simulink model "Multicopter_vPC"  (R2021a)
settings: Solver=ode4  StartTime=0.0  StopTime=inf  FixedStep=0.0002  RelTol=1e-3
values from neighbouring files (symbols this model uses):
  ModelFailBatt_CustomHovTime = 15    [Init.m]
  ModelFailBatt_isEnable = boolean(0)    [Init.m]
  ModelFailBatt_islowCapacity = boolean(0)    [Init.m]
  ModelFailBatt_isLowVoltage = boolean(0)    [Init.m]
  ModelFailBatt_isPowOff = boolean(0)    [Init.m]
  ModelFailBatt_isUseCustomHovTime = boolean(0)    [Init.m]
  ModelFailBatt_remainCapacityRatio = 0.2    [Init.m]
  ModelFailBatt_remainVoltageRatio = 0.5    [Init.m]
  ModelFailEnable = boolean(0)    [Init.m]
  ModelFailLoad_isEnable = boolean(0)    [Init.m]
  ModelFailLoad_isLoadFall = boolean(0)    [Init.m]
  ModelFailLoad_isLoadLeak = boolean(0)    [Init.m]
  ModelFailLoad_isLoadShift = boolean(0)    [Init.m]
  ModelFailLoad_LoadLeakRatioRate = 0    [Init.m]
  ModelFailLoad_loadMassRatio = 0    [Init.m]
  ModelFailLoad_LoadShiftXRatio = 0    [Init.m]
  ModelFailLoad_LoadShiftYRatio = 0    [Init.m]
  ModelFailLoad_LoadShiftZRatio = 0    [Init.m]
  ModelFailProp_isEnable = boolean(1)    [Init.m]
  ModelFailProp_PropEffRatioVec = ones(1,8)    [Init.m]
  ModelFailWind_ConstWindX = 0    [Init.m]
  ModelFailWind_ConstWindY = 0    [Init.m]
  ModelFailWind_ConstWindZ = 0    [Init.m]
  ModelFailWind_GustWindFreq = 0    [Init.m]
  ModelFailWind_GustWindStrength = 0    [Init.m]
  ModelFailWind_isConstWind = boolean(0)    [Init.m]
  ModelFailWind_isEnable = boolean(0)    [Init.m]
  ModelFailWind_isGustWind = boolean(0)    [Init.m]
  ModelFailWind_isSheerWind = boolean(0)    [Init.m]
  ModelFailWind_isTurbWind = boolean(0)    [Init.m]
  ModelFailWind_SheerWindDirec = 0    [Init.m]
  ModelFailWind_SheerWindStrength = 0    [Init.m]
  ModelFailWind_TurbWindDirec = 0    [Init.m]
  ModelFailWind_TurbWindStrength = 0    [Init.m]
  ModelInit_RPM = 0    [Init.m]
  ModelParam_BattHoverMinutes = 18    [Init.m]
  ModelParam_BattHoverThr = 0.609    [Init.m]
  ModelParam_envAltitude = -41.5260009765625    (= -41.5260009766)    [Init.m]
  ModelParam_GlobalNoiseGainSwitch = 0    [Init.m]
  ModelParam_GPSEphFinal = 0.3    [Init.m]
  ModelParam_GPSEpvFinal = 0.4    [Init.m]
  ModelParam_GPSFix3DFix = 3    [Init.m]
  ModelParam_GPSSatsVisible = 10    [Init.m]
  ModelParam_motorCr = 1148    [Init.m]
  ModelParam_motorJm = 0.0001287    [Init.m]
  ModelParam_motorMinThr = 0.05    [Init.m]
  ModelParam_motorT = 0.02    [Init.m]
  ModelParam_motorWb = -141.4    [Init.m]
  ModelParam_noiseBaroCoupleWithSpeed = 0    [Init.m]
  ModelParam_noiseGPSSampTime = 0.2    [Init.m]
  ModelParam_noisePowerIMU = 0    [Init.m]
  ModelParam_noisePowerOffGainAccel = 0.04    [Init.m]
  ModelParam_noisePowerOffGainAccelZ = 0.03    [Init.m]
  ModelParam_noisePowerOffGainGyro = 0.02    [Init.m]
  ModelParam_noisePowerOffGainGyroZ = 0.025    [Init.m]
  ModelParam_noisePowerOffGainMag = 0.02    [Init.m]
  ModelParam_noisePowerOffGainMagZ = 0.035    [Init.m]
  ModelParam_noisePowerOnGainAccel = 0.8    [Init.m]
  ModelParam_noisePowerOnGainAccelZ = 4.5    [Init.m]
  ModelParam_noisePowerOnGainGyro = 2    [Init.m]
  ModelParam_noisePowerOnGainGyroZ = 1    [Init.m]
  ModelParam_noisePowerOnGainMag = 0.025    [Init.m]
  ModelParam_noisePowerOnGainMagZ = 0.05    [Init.m]
  ModelParam_noiseSampleTimeAccel = 0.001    [Init.m]
  ModelParam_noiseSampleTimeGyro = 0.001    [Init.m]
  ModelParam_noiseSampleTimeMag = 0.01    [Init.m]
  ModelParam_noiseUpperBaro = 0    [Init.m]
  ModelParam_noiseUpperGPS = 0.5    [Init.m]
  ModelParam_noiseUpperWindBodyRatio = 0    [Init.m]
  ModelParam_noiseWindSampTime = 0.001    [Init.m]
  ModelParam_rotorCm = 1.779e-07    [Init.m]
  ModelParam_rotorCt = 1.105e-05    [Init.m]
  ModelParam_timeSampBaro = 0.01    [Init.m]
  ModelParam_uavCCm = [0.0035 0.0039 0.0034]    [Init.m]
  ModelParam_uavCd = 0.055    [Init.m]
  ModelParam_uavDearo = 0.12    [Init.m]
  ModelParam_uavJ = [ModelParam_uavJxx,0,0;     0,ModelParam_uavJyy,0;     0,0,ModelParam_uavJzz]    [Init.m]
  ModelParam_uavMass = 1.4    [Init.m]
  ModelParam_uavMotNumbs = int8(4)    [Init.m]
  ModelParam_uavR = 0.225    [Init.m]
  ModelParam_uavType = int8(3)    [Init.m]
undefined symbols (not defined in the file or in its folder): d_i, Earth, F, h_i, Light, MIL, ModelParam_GPSEphInitial, ModelParam_GPSEphTimeConstant, ModelParam_GPSEpvInitial, ModelParam_GPSEpvTimeConstant, ModelParam_noiseLowPassFilterCoeAccel, ModelParam_noiseLowPassFilterCoeGyro, ModelParam_timeSamp, Moderate, Newton, Raphson, WGS84
libraries: simulink x12, aerolibasang x4, aerolibwind2 x3, aerolibtransform2 x3, sharedtransform x3, aerolibutil x2, sharedutil x2, shared6dof x1, aerolibatmos2 x1, aerolibconvert2 x1, aerolibobsolete x1, aerolibnav x1
(part 1 of 3)
settings Model: SimulationMode=accelerator  Creator=Jinrui  LastModifiedBy=YeBobo
settings SolverCC: AlgebraicLoopSolver=TrustRegion
settings DataIOCC: SaveFormat=Structure  SaveOutput=off  SignalLogging=off  DSMLogging=off  SaveTime=off  ReturnWorkspaceOutputs=off
settings DebuggingCC: ParameterTunabilityLossMsg=error  RootOutportRequireBusObject=error  StrictBusMsg=ErrorOnBusTreatedAsVector  SFMachineParentedDataDiag=warning  ArithmeticOperatorsInVariantConditions=warning
settings HardwareCC: ProdBitPerPointer=32  ProdBitPerSizeT=32  ProdBitPerPtrDiffT=32  ProdLargestAtomicFloat=None  ProdWordSize=32  ProdHWDeviceType=Intel->x86/Pentium
settings SFSimCC: SimUseLocalCustomCode=off  CustomCodeUndefinedFunction=UseInterfaceOnly
settings RTWCC: Description=NI Phar Lap Real-Time & Windows Targets  SystemTargetFile=NIVeriStand.tlc  PackageName=MulticopterModel  TemplateMakefile=NIVeriStand_vc.tmf  GenerateReport=on  RTWUseLocalCustomCode=off  LaunchReport=on
settings CodeAppCC: ForceParamTrailComments=on  OperatorAnnotations=on  StateflowObjectComments=on  MATLABSourceComments=on
settings STFCustomTargetCC: TargetLangStandard=C99 (ISO)  MatFileLogging=on  MATLABClassNameForMDSCustomization=Simulink.SoftwareTarget.TargetSpecificTriggerConfigurationBase  UseToolchainInfoCompliant=off  SystemTargetFile=NIVeriStand.tlc
settings GRTTargetCC: ParMdlRefBuildCompliant=off  CompOptLevelCompliant=off  ConcurrentExecutionCompliant=off  CombineOutputUpdateFcns=off  MATLABClassNameForMDSCustomization=Simulink.SoftwareTarget.TargetSpecificTriggerConfigurationBase  CPPClassGenCompliant=off  GRTInterface=on  UseToolchainInfoCompliant=off
settings SimscapeCC: SimscapeNormalizeSystem=off

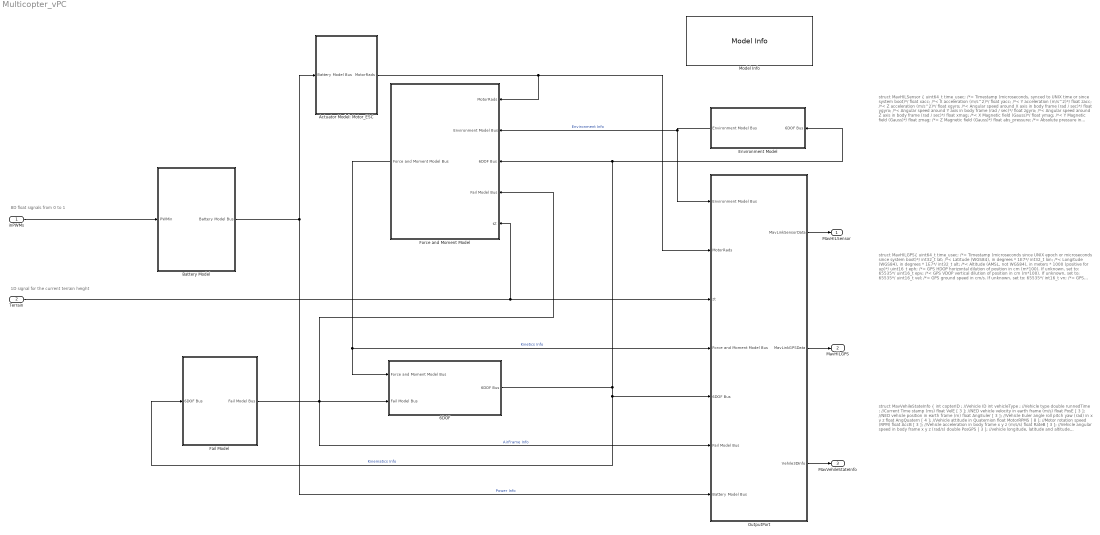
== system Multicopter_vPC ==
  note: struct MavVehileStateInfo {
      | int copterID ; //Vehicle ID
      | int vehicleType ; //Vehicle type
      | double runnedTime ; //Current Time stamp (ms)
      | float VelE [ 3 ]; //NED vehicle velocity in earth frame (m/s)
      | float PosE [ 3 ]; //NED vehicle position in earth frame (m)
      | float AngEuler [ 3 ]; //Vehicle Euler angle roll pitch yaw (rad) in x y z
      | float AngQuatern [ 4 ]; //Vehicle attitude in Quaternion
      | float MotorRPMS [ 8 ]; //Motor rotation speed (RPM)
      | float AccB [ 3 ]; //Vehicle acceleration in body frame x y z (m/s/s)
      | float RateB [ 3 ]; //Vehicle angular speed in body frame x y z (rad/s)
      | double PosGPS [ 3 ]; //vehicle longitude, latitude and altitude (degree,degree,m)
      | }
  note: struct MavHILGPS{
      | uint64_t time_usec; /*< Timestamp (microseconds since UNIX epoch or microseconds since system boot)*/
      | int32_t lat; /*< Latitude (WGS84), in degrees * 1E7*/
      | int32_t lon; /*< Longitude (WGS84), in degrees * 1E7*/
      | int32_t alt; /*< Altitude (AMSL, not WGS84), in meters * 1000 (positive for up)*/
      | uint16_t eph; /*< GPS HDOP horizontal dilution of position in cm (m*100). If unknown, set to: 65535*/
      | uint16_t epv; /*< GPS VDOP vertical dilution of position in cm (m*100). If unknown, set to: 65535*/
      | uint16_t vel; /*< GPS ground speed in cm/s. If unknown, set to: 65535*/
      | int16_t vn; /*< GPS velocity in cm/s in NORTH direction in earth-fixed NED frame*/
      | int16_t ve; /*< GPS velocity in cm/s in EAST direction in earth-fixed NED frame*/
      | int16_t vd; /*< GPS velocity in cm/s in DOWN direction in earth-fixed NED frame*/
      | uint16_t cog; /*< Course over ground (NOT heading, but direction of movement) in degrees * 100, 0.0..359.99 degrees. If unknown, set to: 65535*/
      | uint8_t fix_type; /*< 0-1: no fix, 2: 2D fix, 3: 3D fix. Some applications will not use the value of this field unless it is at least two, so always correctly fill in the fix.*/
      | uint8_t satellites_visible; /*< Number of satellites visible. If unknown, set to 255*/
      | }) ;
  note: struct MavHILSensor {
      | uint64_t time_usec; /*< Timestamp (microseconds, synced to UNIX time or since system boot)*/
      | float xacc; /*< X acceleration (m/s^2)*/
      | float yacc; /*< Y acceleration (m/s^2)*/
      | float zacc; /*< Z acceleration (m/s^2)*/
      | float xgyro; /*< Angular speed around X axis in body frame (rad / sec)*/
      | float ygyro; /*< Angular speed around Y axis in body frame (rad / sec)*/
      | float zgyro; /*< Angular speed around Z axis in body frame (rad / sec)*/
      | float xmag; /*< X Magnetic field (Gauss)*/
      | float ymag; /*< Y Magnetic field (Gauss)*/
      | float zmag; /*< Z Magnetic field (Gauss)*/
      | float abs_pressure; /*< Absolute pressure in millibar*/
      | float diff_pressure; /*< Differential pressure (airspeed) in millibar*/
      | float pressure_alt; /*< Altitude calculated from pressure*/
      | float temperature; /*< Temperature in degrees celsius*/
      | uint32_t fields_updated; /*< Bitmask for fields that have updated since last message, bit 0 = xacc, bit 12: temperature, bit 31: full reset of attitude/position/velocities/etc was performed in sim.*/
      | });
  note: 1D signal for the current terrain height
  note: 8D float signals from 0 to 1
  inPWMs : Inport  PortDimensions=8
  Terrain : Inport  Port=2
  6DOF : Subsystem
  Actuator Model: Motor_ESC : Subsystem
  Battery Model : Subsystem
  Environment Model : Subsystem
  Fail Model : Subsystem
  Force and Moment Model : Subsystem
  Model Info : simulink/Model-Wide Utilities/Model Info  Frame=on  DisplayStringWithTags=|  HorizontalTextAlignment=Center  LeftAlignmentValue=0.5
      | Model Info
      | %<ModelName> 
      | %<Description>   
      | Matlab version is MATLAB R20167. 
      | Coordinate frame is NED frame.
      |  This model  simulates the behavior of multicopters based on performance parameters and RPM inputs
  OutputPort : Subsystem
  MavHILSensor : Outport  OutDataTypeStr=Bus: MavLinkSensor  VectorParamsAs1DForOutWhenUnconnected=off
  MavHILGPS : Outport  Port=2  OutDataTypeStr=Bus: MavLinkGPS  VectorParamsAs1DForOutWhenUnconnected=off
  MavVehileStateInfo : Outport  Port=3  OutDataTypeStr=Bus: MavVehileInfo  VectorParamsAs1DForOutWhenUnconnected=off
  wires:
  OutputPort/3(Vehile3DInfo) -> MavVehileStateInfo/1
  Actuator Model: Motor_ESC/1(MotorRads) -> Force and Moment Model/1(MotorRads), OutputPort/2(MotorRads)
  OutputPort/2(MavLinkGPSData) -> MavHILGPS/1
  Environment Model/1(Environment Model Bus) -> Force and Moment Model/2(Environment Model Bus), OutputPort/1(Environment Model Bus)  "Environment Info"
  Force and Moment Model/1(Force and Moment Model Bus) -> 6DOF/1(Force and Moment Model Bus), OutputPort/4(Force and Moment Model Bus)  "Kinetics Info"
  Fail Model/1(Fail Model Bus) -> OutputPort/6(Fail Model Bus), Force and Moment Model/4(Fail Model Bus), 6DOF/2(Fail Model Bus)  "AirFrame Info"
  inPWMs/1 -> Battery Model/1(PWMin)
  OutputPort/1(MavLinkSensorData) -> MavHILSensor/1
  6DOF/1(6DOF Bus) -> Fail Model/1(6DOF Bus), OutputPort/5(6DOF Bus), Environment Model/1(6DOF Bus), Force and Moment Model/3(6DOF Bus)  "Kinematics Info"
  Terrain/1 -> Force and Moment Model/5("tZ "), OutputPort/3(zt)
  Battery Model/1(Battery Model Bus) -> OutputPort/7(Battery Model Bus), Actuator Model: Motor_ESC/1(Battery Model Bus)  "Power Info"

== system Multicopter_vPC/6DOF ==
  Force and Moment Model Bus : Inport
  Fail Model Bus : Inport  Port=2
  Bus Creator : BusCreator  Inputs=8
  Bus Selector : BusSelector  OutputSignals=dM,m,J
  Bus Selector1 : BusSelector  OutputSignals=Fb,Mb
  Constant_dI/dt : Constant  Value=zeros(3,3)
  Custom Variable Mass 6DOF (Quaternion) : shared6dof/6DOF (Euler Angles)  units=Metric (MKS)  mtype=Custom Variable  rep=Quaternion  xme_0=ModelInit_PosE  Vm_0=ModelInit_VelB  eul_0=ModelInit_AngEuler  pm_0=ModelInit_RateB  mass_0=1.0  mass_e=0.5  mass_f=2.0  inertia=eye(3)  inertia_e=eye(3)  inertia_f=2*eye(3)  k_quat=1.0  vre_flag=off  abi_flag=off  aMode=aMode  xme_statename=''  Vm_statename=''  eul_statename=''  quat_statename=''  pm_statename=''  mass_statename=''
      settings: SourceProductBaseCode=AE,PW,DR,MT,UV,VE
  Sum : Sum  Inputs=++|
  6DOF Bus : Outport  VectorParamsAs1DForOutWhenUnconnected=off
  wires:
  Bus Selector1/1 -> Custom Variable Mass 6DOF (Quaternion)/1  "<Fb>"
  Bus Selector/2 -> Custom Variable Mass 6DOF (Quaternion)/3  "<m>"
  Custom Variable Mass 6DOF (Quaternion)/8 -> Bus Creator/8  "AccB"
  Sum/1 -> Custom Variable Mass 6DOF (Quaternion)/2
  Constant_dI/dt/1 -> Custom Variable Mass 6DOF (Quaternion)/4
  Custom Variable Mass 6DOF (Quaternion)/5 -> Bus Creator/5  "Vb"
  Custom Variable Mass 6DOF (Quaternion)/6 -> Bus Creator/6  "wb"
  Custom Variable Mass 6DOF (Quaternion)/1 -> Bus Creator/1  "Ve"
  Custom Variable Mass 6DOF (Quaternion)/4 -> Bus Creator/4  "DCM"
  Custom Variable Mass 6DOF (Quaternion)/2 -> Bus Creator/2  "Xe"
  Custom Variable Mass 6DOF (Quaternion)/3 -> Bus Creator/3  "Eular(rad)"
  Custom Variable Mass 6DOF (Quaternion)/7 -> Bus Creator/7  "dwb/dt"
  Bus Selector/3 -> Custom Variable Mass 6DOF (Quaternion)/5  "<J>"
  Bus Selector/1 -> Sum/2  "<dM>"
  Bus Selector1/2 -> Sum/1  "<Mb>"
  Fail Model Bus/1 -> Bus Selector/1
  Force and Moment Model Bus/1 -> Bus Selector1/1
  Bus Creator/1 -> 6DOF Bus/1

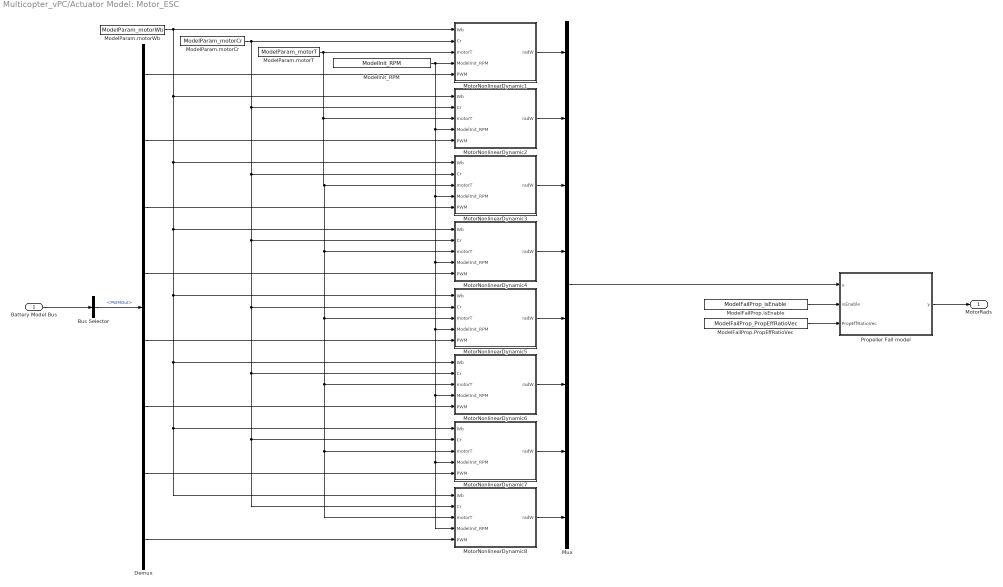
== system Multicopter_vPC/Actuator Model: Motor_ESC ==
  Battery Model Bus : Inport
  Bus Selector : BusSelector  OutputSignals=PWMOut
  Demux : Demux  Outputs=8
  ModelFailProp.PropEffRatioVec : Constant  Value=ModelFailProp_PropEffRatioVec
  ModelFailProp.isEnable : Constant  Value=ModelFailProp_isEnable
  ModelInit_RPM : Constant  Value=ModelInit_RPM
  ModelParam.motorCr : Constant  Value=ModelParam_motorCr
  ModelParam.motorT : Constant  Value=ModelParam_motorT
  ModelParam.motorWb : Constant  Value=ModelParam_motorWb
  MotorNonlinearDynamic1 : Subsystem  TreatAsAtomicUnit=on
  MotorNonlinearDynamic2 : Subsystem  TreatAsAtomicUnit=on
  MotorNonlinearDynamic3 : Subsystem  TreatAsAtomicUnit=on
  MotorNonlinearDynamic4 : Subsystem  TreatAsAtomicUnit=on
  MotorNonlinearDynamic5 : Subsystem  TreatAsAtomicUnit=on
  MotorNonlinearDynamic6 : Subsystem  TreatAsAtomicUnit=on
  MotorNonlinearDynamic7 : Subsystem  TreatAsAtomicUnit=on
  MotorNonlinearDynamic8 : Subsystem  TreatAsAtomicUnit=on
  Mux : Mux  Inputs=8
  Propeller Fail model : MATLAB Function  TreatAsAtomicUnit=on
  MotorRads : Outport  VectorParamsAs1DForOutWhenUnconnected=off
  wires:
  Mux/1 -> Propeller Fail model/1(u)
  Propeller Fail model/1(y) -> MotorRads/1
  ModelFailProp.isEnable/1 -> Propeller Fail model/2(isEnable)
  ModelFailProp.PropEffRatioVec/1 -> Propeller Fail model/3(PropEffRatioVec)
  Demux/1 -> MotorNonlinearDynamic1/5(PWM)
  MotorNonlinearDynamic1/1(radW) -> Mux/1
  Battery Model Bus/1 -> Bus Selector/1
  ModelParam.motorCr/1 -> MotorNonlinearDynamic1/2(Cr), MotorNonlinearDynamic2/2(Cr), MotorNonlinearDynamic3/2(Cr), MotorNonlinearDynamic4/2(Cr), MotorNonlinearDynamic5/2(Cr), MotorNonlinearDynamic6/2(Cr), MotorNonlinearDynamic8/2(Cr), MotorNonlinearDynamic7/2(Cr)
  ModelParam.motorWb/1 -> MotorNonlinearDynamic1/1(Wb), MotorNonlinearDynamic2/1(Wb), MotorNonlinearDynamic3/1(Wb), MotorNonlinearDynamic4/1(Wb), MotorNonlinearDynamic5/1(Wb), MotorNonlinearDynamic6/1(Wb), MotorNonlinearDynamic8/1(Wb), MotorNonlinearDynamic7/1(Wb)
  Demux/2 -> MotorNonlinearDynamic2/5(PWM)
  Demux/3 -> MotorNonlinearDynamic3/5(PWM)
  Demux/4 -> MotorNonlinearDynamic4/5(PWM)
  Demux/5 -> MotorNonlinearDynamic5/5(PWM)
  Demux/6 -> MotorNonlinearDynamic6/5(PWM)
  Demux/7 -> MotorNonlinearDynamic7/5(PWM)
  Demux/8 -> MotorNonlinearDynamic8/5(PWM)
  ModelParam.motorT/1 -> MotorNonlinearDynamic2/3(motorT), MotorNonlinearDynamic3/3(motorT), MotorNonlinearDynamic4/3(motorT), MotorNonlinearDynamic5/3(motorT), MotorNonlinearDynamic6/3(motorT), MotorNonlinearDynamic8/3(motorT), MotorNonlinearDynamic7/3(motorT), MotorNonlinearDynamic1/3(motorT)
  ModelInit_RPM/1 -> MotorNonlinearDynamic2/4(ModelInit_RPM), MotorNonlinearDynamic3/4(ModelInit_RPM), MotorNonlinearDynamic4/4(ModelInit_RPM), MotorNonlinearDynamic5/4(ModelInit_RPM), MotorNonlinearDynamic6/4(ModelInit_RPM), MotorNonlinearDynamic8/4(ModelInit_RPM), MotorNonlinearDynamic7/4(ModelInit_RPM), MotorNonlinearDynamic1/4(ModelInit_RPM)
  MotorNonlinearDynamic2/1(radW) -> Mux/2
  Bus Selector/1 -> Demux/1  "<PWMOut>"
  MotorNonlinearDynamic8/1(radW) -> Mux/8
  MotorNonlinearDynamic7/1(radW) -> Mux/7
  MotorNonlinearDynamic6/1(radW) -> Mux/6
  MotorNonlinearDynamic5/1(radW) -> Mux/5
  MotorNonlinearDynamic4/1(radW) -> Mux/4
  MotorNonlinearDynamic3/1(radW) -> Mux/3

== system Multicopter_vPC/Battery Model ==
  PWMin : Inport
  Bus Creator : BusCreator  Inputs=3
  Clock1 : Clock
  MATLAB Function : MATLAB Function  TreatAsAtomicUnit=on  SystemSampleTime=0.01
  ModelFailBatt.CustomHovTime : Constant  Value=ModelFailBatt_CustomHovTime
  ModelFailBatt.isEnable : Constant  Value=ModelFailBatt_isEnable
  ModelFailBatt.isLowVoltage : Constant  Value=ModelFailBatt_isLowVoltage
  ModelFailBatt.isPowOff : Constant  Value=ModelFailBatt_isPowOff
  ModelFailBatt.isUseCustomHovTime : Constant  Value=ModelFailBatt_isUseCustomHovTime
  ModelFailBatt.islowCapacity : Constant  Value=ModelFailBatt_islowCapacity
  ModelFailBatt.remainCapacityRatio : Constant  Value=ModelFailBatt_remainCapacityRatio
  ModelFailBatt.remainVoltageRatio : Constant  Value=ModelFailBatt_remainVoltageRatio
  ModelParam.BattHoverMinutes : Constant  Value=ModelParam_BattHoverMinutes
  ModelParam.BattHoverThr : Constant  Value=ModelParam_BattHoverThr
  ModelParam.uavMotNumbs : Constant  Value=ModelParam_uavMotNumbs
  Product : Product
  Battery Model Bus : Outport  VectorParamsAs1DForOutWhenUnconnected=off
  wires:
  PWMin/1 -> MATLAB Function/1(load), Product/1  "PWMin"
  MATLAB Function/1(EffRatio) -> Product/2
  ModelParam.BattHoverMinutes/1 -> MATLAB Function/3(hover_time)
  ModelParam.BattHoverThr/1 -> MATLAB Function/4(hover_thr)
  ModelParam.uavMotNumbs/1 -> MATLAB Function/5(motorNumbs)
  MATLAB Function/2(cell_voltage) -> Bus Creator/2  "cellVol"
  Clock1/1 -> MATLAB Function/2(time)
  MATLAB Function/3(remCapacity) -> Bus Creator/3  "remCapa"
  Product/1 -> Bus Creator/1  "PWMOut"
  ModelFailBatt.isEnable/1 -> MATLAB Function/6(isEnable)
  ModelFailBatt.isUseCustomHovTime/1 -> MATLAB Function/7(isUseCustomHovTime)
  ModelFailBatt.CustomHovTime/1 -> MATLAB Function/8(CustomHovTime)
  ModelFailBatt.isPowOff/1 -> MATLAB Function/9(isPowOff)
  ModelFailBatt.isLowVoltage/1 -> MATLAB Function/10(isLowVoltage)
  ModelFailBatt.remainVoltageRatio/1 -> MATLAB Function/11(remainVoltageRatio)
  ModelFailBatt.islowCapacity/1 -> MATLAB Function/12(islowCapacity)
  ModelFailBatt.remainCapacityRatio/1 -> MATLAB Function/13(remainCapacityRatio)
  Bus Creator/1 -> Battery Model Bus/1

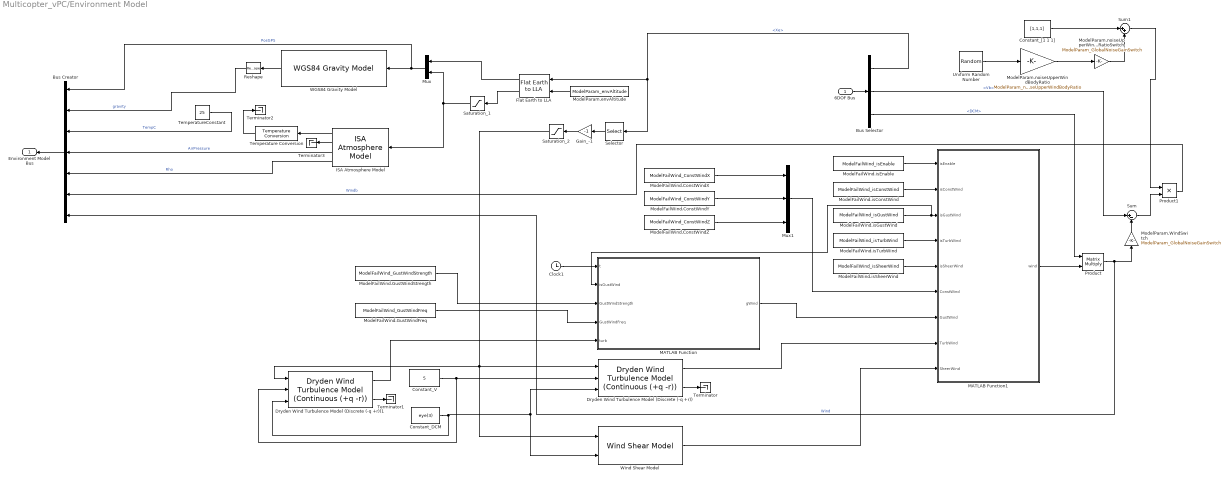
== system Multicopter_vPC/Environment Model ==
  6DOF Bus : Inport
  Bus Creator : BusCreator  Inputs=7
  Bus Selector : BusSelector  OutputSignals=Xe,Vb,DCM
  Clock1 : Clock
  Constant_DCM : Constant  Value=eye(3)
  Constant_V : Constant  Value=5
  Constant_[1 1 1] : Constant  Value=[1,1,1]  VectorParams1D=off
  Dryden Wind Turbulence Model (Discrete (-q +r)) : aerolibwind2/Dryden Wind Turbulence Model  (Continuous (+q -r))  units=Metric (MKS)  spec=MIL-F-8785C  model=Discrete Dryden (-q +r)  W20=ModelFailWind_TurbWindStrength*2.5  Wdeg=ModelFailWind_TurbWindDirec*1  TurbProb=10^-3 - Moderate  L_high=533.4  Wingspan=1  ts=ModelParam_timeSampTurbWind  Seed=[23341 23342 23343 23344]  T_on=on
  Dryden Wind Turbulence Model (Discrete (-q +r))1 : aerolibwind2/Dryden Wind Turbulence Model  (Continuous (+q -r))  units=Metric (MKS)  spec=MIL-F-8785C  model=Discrete Dryden (-q +r)  W20=ModelFailWind_GustWindStrength*1  Wdeg=0  TurbProb=10^-2 - Light  L_high=533.4  Wingspan=1  ts=ModelParam_timeSampTurbWind  Seed=[23301 23542 82443 33344]  T_on=on
  Flat Earth to LLA : aerolibtransform2/Flat Earth to LLA  units=Metric (MKS)  ptype=Earth (WGS84)  F=1/298.257223563  R=6378137  refPosPort=off  LL0=ModelParam_GPSLatLong  psi=0
  Gain_-1 : Gain  Gain=-1
  ISA Atmosphere Model : aerolibatmos2/ISA Atmosphere Model  custom=off  g=9.80665  gamma=1.4  R=287.0531  L=0.0065  h_trop=11000  h_strat=20000  rho0=1.225  P0=101325  T0=288.15  h0=0
  MATLAB Function : MATLAB Function  TreatAsAtomicUnit=on
  MATLAB Function1 : MATLAB Function  TreatAsAtomicUnit=on
  ModelFailWind.ConstWindX : Constant  Value=ModelFailWind_ConstWindX
  ModelFailWind.ConstWindY : Constant  Value=ModelFailWind_ConstWindY
  ModelFailWind.ConstWindZ : Constant  Value=ModelFailWind_ConstWindZ
  ModelFailWind.GustWindFreq : Constant  Value=ModelFailWind_GustWindFreq
  ModelFailWind.GustWindStrength : Constant  Value=ModelFailWind_GustWindStrength
  ModelFailWind.isConstWind : Constant  Value=ModelFailWind_isConstWind
  ModelFailWind.isEnable : Constant  Value=ModelFailWind_isEnable
  ModelFailWind.isGustWind : Constant  Value=ModelFailWind_isGustWind
  ModelFailWind.isSheerWind : Constant  Value=ModelFailWind_isSheerWind
  ModelFailWind.isTurbWind : Constant  Value=ModelFailWind_isTurbWind
  ModelParam.WindSwitch : Gain  Gain=ModelParam_GlobalNoiseGainSwitch
  ModelParam.envAltitude : Constant  Value=ModelParam_envAltitude
  ModelParam.noiseUpperWindBodyRatio : Gain  Gain=ModelParam_noiseUpperWindBodyRatio
  ModelParam.noiseUpperWindBodyRatioSwitch : Gain  Gain=ModelParam_GlobalNoiseGainSwitch
  Mux : Mux  Inputs=2
  Mux1 : Mux  Inputs=3
  Product : Product  Multiplication=Matrix(*)
  Product1 : Product
  Reshape : Reshape
  Saturation_1 : Saturate  UpperLimit=100000  LowerLimit=0
  Saturation_2 : Saturate  UpperLimit=10000  LowerLimit=0
  Selector : Selector  InputPortWidth=3  IndexOptions=Index vector (dialog)  Indices=[3]  OutputSizes=1
  Sum : Sum  Inputs=|+-
  Sum1 : Sum  Inputs=|++
  Temperature Conversion : aerolibconvert2/Temperature Conversion  IU=K  OU=C
      settings: SourceProductBaseCode=AE
  TemperatureConstant : Constant  Value=25
  Terminator{,1..3} (4 alike) : Terminator
  Uniform Random Number : UniformRandomNumber  Minimum=[-1,-1,-0.5]  Maximum=[1,1,0.5]  Seed=[564565,6846798,46545]  SampleTime=ModelParam_noiseWindSampTime
  "WGS84 Gravity Model " : aerolibobsolete/WGS84 Gravity Model   model=WGS84 Taylor Series  units=Metric (MKS)  no_atmos=on  precessing=on  jd_loc=off  month=October  day=10  year=2004  no_centrifugal=on  action=Warning
      settings: SourceProductBaseCode=AE
  Wind Shear Model : aerolibwind2/Wind Shear Model  units=Metric (MKS)  phase=Category C - Terminal Flight Phase  W_20=ModelFailWind_SheerWindStrength*1  Wdeg=ModelFailWind_SheerWindDirec*1
  Environment Model Bus : Outport  VectorParamsAs1DForOutWhenUnconnected=off
  wires:
  "WGS84 Gravity Model "/1 -> Reshape/1
  Reshape/1 -> Bus Creator/2  "gravity"
  ISA Atmosphere Model/1 -> Temperature Conversion/1
  ISA Atmosphere Model/2 -> Terminator3/1
  ISA Atmosphere Model/3 -> Bus Creator/4  "AirPressure"
  ISA Atmosphere Model/4 -> Bus Creator/5  "Rho"
  Flat Earth to LLA/2 -> Saturation_1/1
  Saturation_1/1 -> Mux/2, ISA Atmosphere Model/1
  ModelParam.envAltitude/1 -> Flat Earth to LLA/2
  Mux/1 -> Bus Creator/1, "WGS84 Gravity Model "/1  "PosGPS"
  Flat Earth to LLA/1 -> Mux/1
  Clock1/1 -> MATLAB Function/1(t)
  MATLAB Function/1(gWind) -> MATLAB Function1/7(GustWind)
  Dryden Wind Turbulence Model (Discrete (-q +r))/2 -> Terminator/1
  Dryden Wind Turbulence Model (Discrete (-q +r))/1 -> MATLAB Function1/8(TurbWind)
  Constant_DCM/1 -> Dryden Wind Turbulence Model (Discrete (-q +r))/3, Wind Shear Model/2, Dryden Wind Turbulence Model (Discrete (-q +r))1/3
  Constant_V/1 -> Dryden Wind Turbulence Model (Discrete (-q +r))1/2, Dryden Wind Turbulence Model (Discrete (-q +r))/2
  Selector/1 -> Gain_-1/1
  Gain_-1/1 -> Saturation_2/1
  Saturation_2/1 -> Dryden Wind Turbulence Model (Discrete (-q +r))/1, Wind Shear Model/1, Dryden Wind Turbulence Model (Discrete (-q +r))1/1
  MATLAB Function1/1(wind) -> Product/2
  Mux1/1 -> MATLAB Function1/6(ConstWind)
  Wind Shear Model/1 -> MATLAB Function1/9(SheerWind)
  Dryden Wind Turbulence Model (Discrete (-q +r))1/2 -> Terminator1/1
  Bus Selector/3 -> Product/1  "<DCM>"
  Bus Selector/2 -> Sum/1  "<Vb>"
  Product/1 -> Bus Creator/7, ModelParam.WindSwitch/1  "Wind"
  Uniform Random Number/1 -> ModelParam.noiseUpperWindBodyRatio/1
  Sum/1 -> Product1/2
  Product1/1 -> Bus Creator/6  "Windb"
  Constant_[1 1 1]/1 -> Sum1/1
  ModelParam.noiseUpperWindBodyRatio/1 -> ModelParam.noiseUpperWindBodyRatioSwitch/1
  Sum1/1 -> Product1/1
  ModelFailWind.isEnable/1 -> MATLAB Function1/1(isEnable)
  ModelFailWind.isConstWind/1 -> MATLAB Function1/2(isConstWind)
  ModelFailWind.isGustWind/1 -> MATLAB Function/2(isGustWind), MATLAB Function1/3(isGustWind)
  ModelFailWind.GustWindFreq/1 -> MATLAB Function/4(GustWindFreq)
  ModelFailWind.isTurbWind/1 -> MATLAB Function1/4(isTurbWind)
  ModelFailWind.isSheerWind/1 -> MATLAB Function1/5(isSheerWind)
  Dryden Wind Turbulence Model (Discrete (-q +r))1/1 -> MATLAB Function/5(turb)
  ModelFailWind.GustWindStrength/1 -> MATLAB Function/3(GustWindStrength)
  Temperature Conversion/1 -> Terminator2/1
  TemperatureConstant/1 -> Bus Creator/3  "TempC"
  ModelFailWind.ConstWindX/1 -> Mux1/1
  ModelFailWind.ConstWindY/1 -> Mux1/2
  ModelFailWind.ConstWindZ/1 -> Mux1/3
  ModelParam.WindSwitch/1 -> Sum/2
  ModelParam.noiseUpperWindBodyRatioSwitch/1 -> Sum1/2
  6DOF Bus/1 -> Bus Selector/1
  Bus Selector/1 -> Selector/1, Flat Earth to LLA/1  "<Xe>"
  Bus Creator/1 -> Environment Model Bus/1

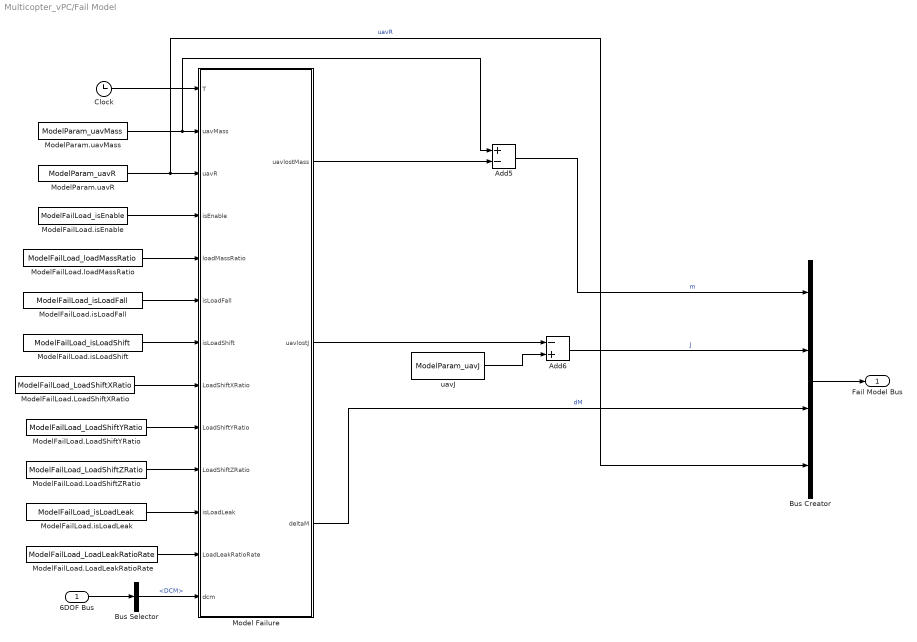
== system Multicopter_vPC/Fail Model ==
  6DOF Bus : Inport
  Add5 : Sum  Inputs=+-
  Add6 : Sum  Inputs=-+
  Bus Creator : BusCreator  Inputs=4
  Bus Selector : BusSelector  OutputSignals=DCM
  Clock : Clock
  Model Failure : MATLAB Function  TreatAsAtomicUnit=on
  ModelFailLoad.LoadLeakRatioRate : Constant  Value=ModelFailLoad_LoadLeakRatioRate
  ModelFailLoad.LoadShiftXRatio : Constant  Value=ModelFailLoad_LoadShiftXRatio
  ModelFailLoad.LoadShiftYRatio : Constant  Value=ModelFailLoad_LoadShiftYRatio
  ModelFailLoad.LoadShiftZRatio : Constant  Value=ModelFailLoad_LoadShiftZRatio
  ModelFailLoad.isEnable : Constant  Value=ModelFailLoad_isEnable
  ModelFailLoad.isLoadFall : Constant  Value=ModelFailLoad_isLoadFall
  ModelFailLoad.isLoadLeak : Constant  Value=ModelFailLoad_isLoadLeak
  ModelFailLoad.isLoadShift : Constant  Value=ModelFailLoad_isLoadShift
  ModelFailLoad.loadMassRatio : Constant  Value=ModelFailLoad_loadMassRatio
  ModelParam.uavMass : Constant  Value=ModelParam_uavMass
  ModelParam.uavR : Constant  Value=ModelParam_uavR
  uavJ : Constant  Value=ModelParam_uavJ
  Fail Model Bus : Outport  VectorParamsAs1DForOutWhenUnconnected=off
  wires:
  Add6/1 -> Bus Creator/2  "J"
  Add5/1 -> Bus Creator/1  "m"
  uavJ/1 -> Add6/2
  ModelParam.uavMass/1 -> Add5/1, Model Failure/2(uavMass)
  ModelParam.uavR/1 -> Bus Creator/4, Model Failure/3(uavR)  "uavR"
  Model Failure/1(uavlostMass) -> Add5/2
  Model Failure/2(uavlostJ) -> Add6/1
  Clock/1 -> Model Failure/1(T)
  Model Failure/3(deltaM) -> Bus Creator/3  "dM"
  ModelFailLoad.LoadLeakRatioRate/1 -> Model Failure/12(LoadLeakRatioRate)
  ModelFailLoad.isLoadLeak/1 -> Model Failure/11(isLoadLeak)
  ModelFailLoad.LoadShiftZRatio/1 -> Model Failure/10(LoadShiftZRatio)
  ModelFailLoad.LoadShiftYRatio/1 -> Model Failure/9(LoadShiftYRatio)
  ModelFailLoad.LoadShiftXRatio/1 -> Model Failure/8(LoadShiftXRatio)
  ModelFailLoad.isLoadShift/1 -> Model Failure/7(isLoadShift)
  ModelFailLoad.isLoadFall/1 -> Model Failure/6(isLoadFall)
  ModelFailLoad.loadMassRatio/1 -> Model Failure/5(loadMassRatio)
  ModelFailLoad.isEnable/1 -> Model Failure/4(isEnable)
  Bus Creator/1 -> Fail Model Bus/1
  6DOF Bus/1 -> Bus Selector/1
  Bus Selector/1 -> Model Failure/13(dcm)  "<DCM>"

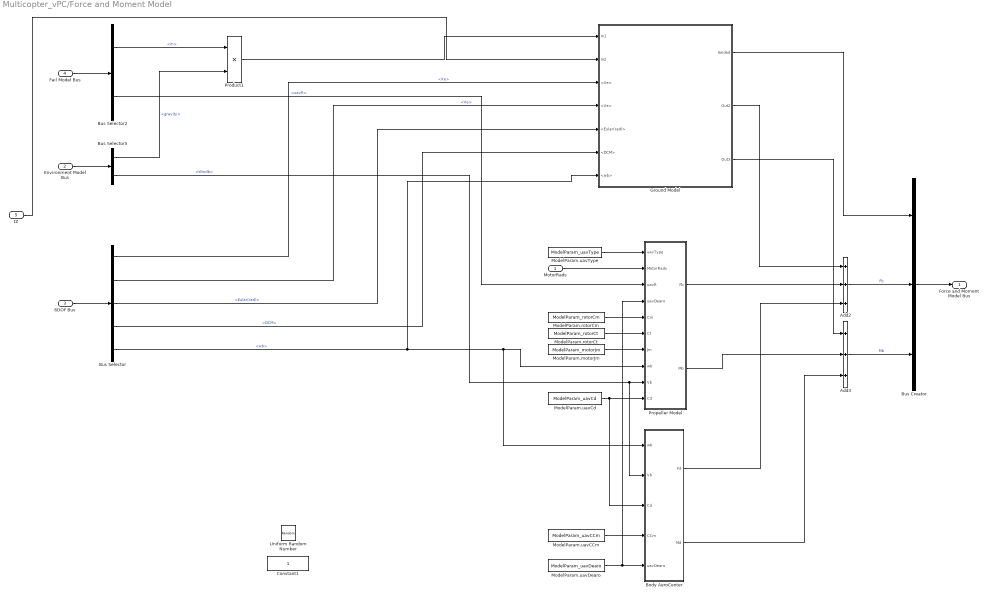
== system Multicopter_vPC/Force and Moment Model ==
  MotorRads : Inport
  Environment Model Bus : Inport  Port=2
  6DOF Bus : Inport  Port=3
  Fail Model Bus : Inport  Port=4
  "tZ " : Inport  Port=5
  Add2 : Sum  Inputs=+++
  Add3 : Sum  Inputs=+++
  Body AeroCenter : MATLAB Function  TreatAsAtomicUnit=on
  Bus Creator : BusCreator  Inputs=3
  Bus Selector : BusSelector  OutputSignals=Xe,Ve,Eular(rad),DCM,wb
  Bus Selector2 : BusSelector  OutputSignals=m,uavR
  Bus Selector5 : BusSelector  OutputSignals=gravity,Windb
  Constant1 : Constant
  Ground Model : Subsystem
  ModelParam.motorJm : Constant  Value=ModelParam_motorJm
  ModelParam.rotorCm : Constant  Value=ModelParam_rotorCm
  ModelParam.rotorCt : Constant  Value=ModelParam_rotorCt
  ModelParam.uavCCm : Constant  Value=ModelParam_uavCCm
  ModelParam.uavCd : Constant  Value=ModelParam_uavCd
  ModelParam.uavDearo : Constant  Value=ModelParam_uavDearo
  ModelParam.uavType : Constant  Value=ModelParam_uavType
  Product1 : Product
  Propeller Model : Subsystem  TreatAsAtomicUnit=on
  Uniform Random Number : UniformRandomNumber  Minimum=[-1,-1,-1]  Maximum=[1,1,1]  Seed=[145787,351545,2864]  SampleTime=0.05
  Force and Moment Model Bus : Outport  VectorParamsAs1DForOutWhenUnconnected=off
  wires:
  Body AeroCenter/2(Md) -> Add3/3
  Body AeroCenter/1(Fd) -> Add2/3
  Propeller Model/2(Mb) -> Add3/2
  Propeller Model/1(Fb) -> Add2/2
  Add3/1 -> Bus Creator/3  "Mb"
  Add2/1 -> Bus Creator/2  "Fb"
  ModelParam.uavType/1 -> Propeller Model/1(uavType)
  ModelParam.rotorCt/1 -> Propeller Model/6(Ct)
  ModelParam.uavCd/1 -> Propeller Model/10(Cd), Body AeroCenter/3(Cd)
  ModelParam.motorJm/1 -> Propeller Model/7(Jm)
  ModelParam.rotorCm/1 -> Propeller Model/5(Cm)
  MotorRads/1 -> Propeller Model/2(MotorRads)
  Bus Selector/5 -> Ground Model/7(<wb>), Propeller Model/8(wb), Body AeroCenter/1(wb)  "<wb>"
  ModelParam.uavCCm/1 -> Body AeroCenter/4(CCm)
  Bus Creator/1 -> Force and Moment Model Bus/1
  6DOF Bus/1 -> Bus Selector/1
  Bus Selector2/1 -> Product1/1  "<m>"
  Bus Selector5/1 -> Product1/2  "<gravity>"
  Fail Model Bus/1 -> Bus Selector2/1
  Environment Model Bus/1 -> Bus Selector5/1
  Bus Selector2/2 -> Propeller Model/3(uavR)  "<uavR>"
  Bus Selector5/2 -> Propeller Model/9(Vb), Body AeroCenter/2(Vb)  "<Windb>"
  ModelParam.uavDearo/1 -> Propeller Model/4(uavDearo), Body AeroCenter/5(uavDearo)
  Product1/1 -> Ground Model/1(In1)
  "tZ "/1 -> Ground Model/2(In2)
  Bus Selector/1 -> Ground Model/3(<Xe>)  "<Xe>"
  Bus Selector/2 -> Ground Model/4(<Ve>)  "<Ve>"
  Bus Selector/3 -> Ground Model/5(<Eular(rad)>)  "<Eular(rad)>"
  Bus Selector/4 -> Ground Model/6(<DCM>)  "<DCM>"
  Ground Model/1(landed) -> Bus Creator/1
  Ground Model/2(Out2) -> Add2/1
  Ground Model/3(Out3) -> Add3/1

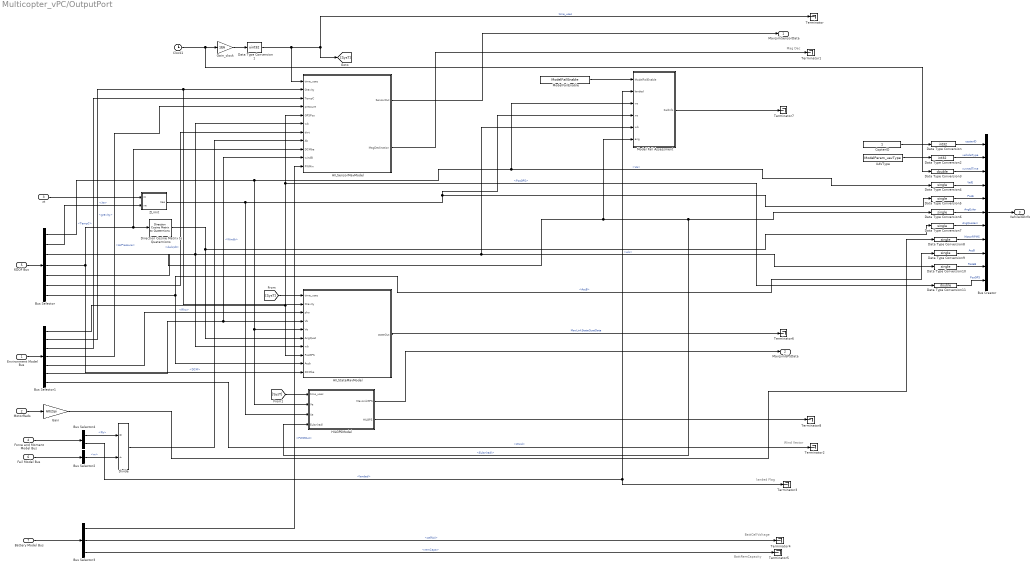
== system Multicopter_vPC/OutputPort ==
  note: Mag Dec
  note: Wind Vector
  note: landed Flag
  note: BattRemCapacity
  note: BattCellVoltage
  Environment Model Bus : Inport
  MotorRads : Inport  Port=2
  zt : Inport  Port=3
  Force and Moment Model Bus : Inport  Port=4
  6DOF Bus : Inport  Port=5
  Fail Model Bus : Inport  Port=6
  Battery Model Bus : Inport  Port=7
  Bus Creator : BusCreator  Inputs=11  OutDataTypeStr=Bus: MavVehileInfo
  Bus Selector : BusSelector  OutputSignals=Ve,Xe,Eular(rad),DCM,wb,dwb/dt,AccB
  Bus Selector1 : BusSelector  OutputSignals=PosGPS,gravity,TempC,AirPressure,Rho,Windb,Wind
  Bus Selector2 : BusSelector  OutputSignals=m
  Bus Selector3 : BusSelector  OutputSignals=PWMOut,cellVol,remCapa
  Bus Selector4 : BusSelector  OutputSignals=Fb,landed
  Clock1 : Clock
  CopterID : Constant
  Data Type Conversion : DataTypeConversion  OutDataTypeStr=int32
  Data Type Conversion1 : DataTypeConversion  OutDataTypeStr=uint32
  Data Type Conversion{4..10} (7 alike) : DataTypeConversion  OutDataTypeStr=single
  Data Type Conversion11 : DataTypeConversion  OutDataTypeStr=double
  Data Type Conversion2 : DataTypeConversion  OutDataTypeStr=int32
  Data Type Conversion3 : DataTypeConversion  OutDataTypeStr=double
  Direction Cosine Matrix to Quaternions : sharedtransform/Direction Cosine Matrix  to Quaternions  aMode=aMode  action=None  tolerance=eps(2)
      settings: SourceProductBaseCode=AE,PW,DR,MT,UV,VE
  Divide : Product  Inputs=*/
  Gain : Gain  Gain=60/2/pi
  Gain_clock : Gain  Gain=1E6
  HILGPSModel : Subsystem
  HILSensorMavModel : Subsystem
  HILStateMavModel : Subsystem
  Model Fail Assessment : MATLAB Function  TreatAsAtomicUnit=on
  ModelFailEnable : Constant  Value=ModelFailEnable
  Terminator{,1..8} (9 alike) : Terminator
  UAVType : Constant  Value=ModelParam_uavType
  ZLimit : MATLAB Function  TreatAsAtomicUnit=on
  MavLinkSensorData : Outport  VectorParamsAs1DForOutWhenUnconnected=off
  MavLinkGPSData : Outport  Port=2  VectorParamsAs1DForOutWhenUnconnected=off
  Vehile3DInfo : Outport  Port=3  VectorParamsAs1DForOutWhenUnconnected=off
  wires:
  [SysT] -> HILGPSModel/1(time_usec)
  [SysT] -> HILStateMavModel/1(time_usec)
  Bus Selector/5 -> HILSensorMavModel/6(wb), Data Type Conversion10/1, Model Fail Assessment/5(wb), HILStateMavModel/7(wb)  "<wb>"
  Bus Selector/4 -> HILStateMavModel/10(DCMbe), HILSensorMavModel/9(DCMbe), Direction Cosine Matrix to Quaternions/1  "<DCM>"
  Bus Selector/1 -> HILGPSModel/2(Ve), HILStateMavModel/5(Ve), Model Fail Assessment/3(ve), Data Type Conversion4/1  "<Ve>"
  Bus Selector/6 -> HILSensorMavModel/7(dwt)  "<dwb/dt>"
  Bus Selector/3 -> Data Type Conversion6/1, HILGPSModel/4(Eular(rad)), Model Fail Assessment/6(ang)  "<Eular(rad)>"
  Clock1/1 -> Data Type Conversion3/1, Gain_clock/1
  Data Type Conversion1/1 -> HILSensorMavModel/1(time_usec), Terminator/1, [SysT]  "time_usec"
  Gain_clock/1 -> Data Type Conversion1/1
  ModelFailEnable/1 -> Model Fail Assessment/1(ModelFailEnable)
  6DOF Bus/1 -> Bus Selector/1
  zt/1 -> ZLimit/1(zt)
  Bus Selector/2 -> ZLimit/2(xe)  "<Xe>"
  Environment Model Bus/1 -> Bus Selector1/1
  Bus Selector1/1 -> Data Type Conversion11/1, HILSensorMavModel/5(GPSPos), HILStateMavModel/8(PosGPS)  "<PosGPS>"
  Bus Selector1/2 -> HILStateMavModel/2(Gravity), HILSensorMavModel/2(Gravity)  "<gravity>"
  Bus Selector1/3 -> HILSensorMavModel/3(TempC)  "<TempC>"
  Bus Selector1/4 -> HILSensorMavModel/4(pressure)  "<AirPressure>"
  Bus Selector1/5 -> HILStateMavModel/3(pho)  "<Rho>"
  Bus Selector1/6 -> HILSensorMavModel/10(windB), HILStateMavModel/4(Vb)  "<Windb>"
  Bus Selector2/1 -> Divide/2  "<m>"
  Bus Selector4/1 -> Divide/1  "<Fb>"
  Force and Moment Model Bus/1 -> Bus Selector4/1
  Fail Model Bus/1 -> Bus Selector2/1
  Bus Selector4/2 -> Model Fail Assessment/2(landed), Terminator3/1  "<landed>"
  Battery Model Bus/1 -> Bus Selector3/1
  Bus Selector3/2 -> Terminator4/1  "<cellVol>"
  Bus Selector3/3 -> Terminator5/1  "<remCapa>"
  Bus Selector3/1 -> HILSensorMavModel/11(PWMin)  "<PWMOut>"
  Bus Selector1/7 -> Terminator2/1  "<Wind>"
  MotorRads/1 -> Gain/1
  HILSensorMavModel/1(SensorOut) -> MavLinkSensorData/1
  HILSensorMavModel/2(MagDeclination) -> Terminator1/1
  Model Fail Assessment/1(FailInfo) -> Terminator7/1
  ZLimit/1(Xee) -> Data Type Conversion5/1, Model Fail Assessment/4(xe), HILGPSModel/3(Xe)
  Direction Cosine Matrix to Quaternions/1 -> Data Type Conversion7/1, HILStateMavModel/6(AngQuat)
  Divide/1 -> HILSensorMavModel/8(Ab)
  HILStateMavModel/1(stateOut) -> Terminator6/1  "MavLinkStateQuatData"
  HILGPSModel/1(MavLinkGPS) -> MavLinkGPSData/1
  HILGPSModel/2(HILGPS) -> Terminator8/1
  Gain/1 -> Data Type Conversion8/1
  Bus Selector/7 -> Data Type Conversion9/1, HILStateMavModel/9(Accb)  "<AccB>"
  CopterID/1 -> Data Type Conversion/1
  Data Type Conversion/1 -> Bus Creator/1  "copterID"
  Data Type Conversion2/1 -> Bus Creator/2  "vehicleType"
  UAVType/1 -> Data Type Conversion2/1
  Data Type Conversion3/1 -> Bus Creator/3  "runnedTime"
  Data Type Conversion4/1 -> Bus Creator/4  "VelE"
  Data Type Conversion5/1 -> Bus Creator/5  "PosE"
  Data Type Conversion6/1 -> Bus Creator/6  "AngEuler"
  Data Type Conversion7/1 -> Bus Creator/7  "AngQuatern"
  Data Type Conversion8/1 -> Bus Creator/8  "MotorRPMS"
  Data Type Conversion9/1 -> Bus Creator/9  "AccB"
  Data Type Conversion10/1 -> Bus Creator/10  "RateB"
  Data Type Conversion11/1 -> Bus Creator/11  "PosGPS"
  Bus Creator/1 -> Vehile3DInfo/1

== system Multicopter_vPC/Actuator Model: Motor_ESC/MotorNonlinearDynamic1 ==
  Wb : Inport
  Cr : Inport  Port=2
  motorT : Inport  Port=3
  ModelInit_RPM : Inport  Port=4
  PWM : Inport  Port=5
  Minimum Throttle Cutoff : simulink/Logic and Bit Operations/Compare To Constant  relop=>=  const=ModelParam_motorMinThr  OutDataTypeStr=uint8
  Motor_Dynamics : Subsystem  TreatAsAtomicUnit=on
  Motor_Dynamics_backup : StateSpace  Commented=on  A=-1/ModelParam_motorT  C=1/ModelParam_motorT  D=0  InitialCondition=ModelInit_RPM*ModelParam_motorT
  Product : Product
  Product1 : Product
  Signal_Saturation : Saturate  UpperLimit=0.95  LowerLimit=0
  Sum1 : Sum  Inputs=++|
  radW : Outport  VectorParamsAs1DForOutWhenUnconnected=off
  wires:
  PWM/1 -> Signal_Saturation/1
  Motor_Dynamics/1(motor_rate_act) -> radW/1
  Product/1 -> Motor_Dynamics/1(motor_rate_d)
  Signal_Saturation/1 -> Product1/2, Minimum Throttle Cutoff/1
  Product1/1 -> Sum1/2
  Sum1/1 -> Product/1
  Wb/1 -> Sum1/1
  Minimum Throttle Cutoff/1 -> Product/2
  Cr/1 -> Product1/1
  motorT/1 -> Motor_Dynamics/3(motorT)
  ModelInit_RPM/1 -> Motor_Dynamics/2(ModelInit_RPM)

== system Multicopter_vPC/Actuator Model: Motor_ESC/MotorNonlinearDynamic2 ==
  Wb : Inport
  Cr : Inport  Port=2
  motorT : Inport  Port=3
  ModelInit_RPM : Inport  Port=4
  PWM : Inport  Port=5
  Minimum Throttle Cutoff : simulink/Logic and Bit Operations/Compare To Constant  relop=>=  const=ModelParam_motorMinThr  OutDataTypeStr=uint8
  Motor_Dynamics : Subsystem  TreatAsAtomicUnit=on
  Motor_Dynamics_backup : StateSpace  Commented=on  A=-1/ModelParam_motorT  C=1/ModelParam_motorT  D=0  InitialCondition=ModelInit_RPM*ModelParam_motorT
  Product : Product
  Product1 : Product
  Signal_Saturation : Saturate  UpperLimit=0.95  LowerLimit=0
  Sum1 : Sum  Inputs=++|
  radW : Outport  VectorParamsAs1DForOutWhenUnconnected=off
  wires:
  ModelInit_RPM/1 -> Motor_Dynamics/2(ModelInit_RPM)
  motorT/1 -> Motor_Dynamics/3(motorT)
  Cr/1 -> Product1/1
  Minimum Throttle Cutoff/1 -> Product/2
  Wb/1 -> Sum1/1
  Sum1/1 -> Product/1
  Product1/1 -> Sum1/2
  Signal_Saturation/1 -> Minimum Throttle Cutoff/1, Product1/2
  Product/1 -> Motor_Dynamics/1(motor_rate_d)
  Motor_Dynamics/1(motor_rate_act) -> radW/1
  PWM/1 -> Signal_Saturation/1

== system Multicopter_vPC/Actuator Model: Motor_ESC/MotorNonlinearDynamic3 ==
  Wb : Inport
  Cr : Inport  Port=2
  motorT : Inport  Port=3
  ModelInit_RPM : Inport  Port=4
  PWM : Inport  Port=5
  Minimum Throttle Cutoff : simulink/Logic and Bit Operations/Compare To Constant  relop=>=  const=ModelParam_motorMinThr  OutDataTypeStr=uint8
  Motor_Dynamics : Subsystem  TreatAsAtomicUnit=on
  Motor_Dynamics_backup : StateSpace  Commented=on  A=-1/ModelParam_motorT  C=1/ModelParam_motorT  D=0  InitialCondition=ModelInit_RPM*ModelParam_motorT
  Product : Product
  Product1 : Product
  Signal_Saturation : Saturate  UpperLimit=0.95  LowerLimit=0
  Sum1 : Sum  Inputs=++|
  radW : Outport  VectorParamsAs1DForOutWhenUnconnected=off
  wires:
  PWM/1 -> Signal_Saturation/1
  Motor_Dynamics/1(motor_rate_act) -> radW/1
  Product/1 -> Motor_Dynamics/1(motor_rate_d)
  Signal_Saturation/1 -> Product1/2, Minimum Throttle Cutoff/1
  Product1/1 -> Sum1/2
  Sum1/1 -> Product/1
  Wb/1 -> Sum1/1
  Minimum Throttle Cutoff/1 -> Product/2
  Cr/1 -> Product1/1
  motorT/1 -> Motor_Dynamics/3(motorT)
  ModelInit_RPM/1 -> Motor_Dynamics/2(ModelInit_RPM)

== system Multicopter_vPC/Actuator Model: Motor_ESC/MotorNonlinearDynamic4 ==
  Wb : Inport
  Cr : Inport  Port=2
  motorT : Inport  Port=3
  ModelInit_RPM : Inport  Port=4
  PWM : Inport  Port=5
  Minimum Throttle Cutoff : simulink/Logic and Bit Operations/Compare To Constant  relop=>=  const=ModelParam_motorMinThr  OutDataTypeStr=uint8
  Motor_Dynamics : Subsystem  TreatAsAtomicUnit=on
  Motor_Dynamics_backup : StateSpace  Commented=on  A=-1/ModelParam_motorT  C=1/ModelParam_motorT  D=0  InitialCondition=ModelInit_RPM*ModelParam_motorT
  Product : Product
  Product1 : Product
  Signal_Saturation : Saturate  UpperLimit=0.95  LowerLimit=0
  Sum1 : Sum  Inputs=++|
  radW : Outport  VectorParamsAs1DForOutWhenUnconnected=off
  wires:
  ModelInit_RPM/1 -> Motor_Dynamics/2(ModelInit_RPM)
  motorT/1 -> Motor_Dynamics/3(motorT)
  Cr/1 -> Product1/1
  Minimum Throttle Cutoff/1 -> Product/2
  Wb/1 -> Sum1/1
  Sum1/1 -> Product/1
  Product1/1 -> Sum1/2
  Signal_Saturation/1 -> Minimum Throttle Cutoff/1, Product1/2
  Product/1 -> Motor_Dynamics/1(motor_rate_d)
  Motor_Dynamics/1(motor_rate_act) -> radW/1
  PWM/1 -> Signal_Saturation/1

== system Multicopter_vPC/Actuator Model: Motor_ESC/MotorNonlinearDynamic5 ==
  Wb : Inport
  Cr : Inport  Port=2
  motorT : Inport  Port=3
  ModelInit_RPM : Inport  Port=4
  PWM : Inport  Port=5
  Minimum Throttle Cutoff : simulink/Logic and Bit Operations/Compare To Constant  relop=>=  const=ModelParam_motorMinThr  OutDataTypeStr=uint8
  Motor_Dynamics : Subsystem  TreatAsAtomicUnit=on
  Motor_Dynamics_backup : StateSpace  Commented=on  A=-1/ModelParam_motorT  C=1/ModelParam_motorT  D=0  InitialCondition=ModelInit_RPM*ModelParam_motorT
  Product : Product
  Product1 : Product
  Signal_Saturation : Saturate  UpperLimit=0.95  LowerLimit=0
  Sum1 : Sum  Inputs=++|
  radW : Outport  VectorParamsAs1DForOutWhenUnconnected=off
  wires:
  PWM/1 -> Signal_Saturation/1
  Motor_Dynamics/1(motor_rate_act) -> radW/1
  Product/1 -> Motor_Dynamics/1(motor_rate_d)
  Signal_Saturation/1 -> Product1/2, Minimum Throttle Cutoff/1
  Product1/1 -> Sum1/2
  Sum1/1 -> Product/1
  Wb/1 -> Sum1/1
  Minimum Throttle Cutoff/1 -> Product/2
  Cr/1 -> Product1/1
  motorT/1 -> Motor_Dynamics/3(motorT)
  ModelInit_RPM/1 -> Motor_Dynamics/2(ModelInit_RPM)

== system Multicopter_vPC/Actuator Model: Motor_ESC/MotorNonlinearDynamic6 ==
  Wb : Inport
  Cr : Inport  Port=2
  motorT : Inport  Port=3
  ModelInit_RPM : Inport  Port=4
  PWM : Inport  Port=5
  Minimum Throttle Cutoff : simulink/Logic and Bit Operations/Compare To Constant  relop=>=  const=ModelParam_motorMinThr  OutDataTypeStr=uint8
  Motor_Dynamics : Subsystem  TreatAsAtomicUnit=on
  Motor_Dynamics_backup : StateSpace  Commented=on  A=-1/ModelParam_motorT  C=1/ModelParam_motorT  D=0  InitialCondition=ModelInit_RPM*ModelParam_motorT
  Product : Product
  Product1 : Product
  Signal_Saturation : Saturate  UpperLimit=0.95  LowerLimit=0
  Sum1 : Sum  Inputs=++|
  radW : Outport  VectorParamsAs1DForOutWhenUnconnected=off
  wires:
  ModelInit_RPM/1 -> Motor_Dynamics/2(ModelInit_RPM)
  motorT/1 -> Motor_Dynamics/3(motorT)
  Cr/1 -> Product1/1
  Minimum Throttle Cutoff/1 -> Product/2
  Wb/1 -> Sum1/1
  Sum1/1 -> Product/1
  Product1/1 -> Sum1/2
  Signal_Saturation/1 -> Minimum Throttle Cutoff/1, Product1/2
  Product/1 -> Motor_Dynamics/1(motor_rate_d)
  Motor_Dynamics/1(motor_rate_act) -> radW/1
  PWM/1 -> Signal_Saturation/1

== system Multicopter_vPC/Actuator Model: Motor_ESC/MotorNonlinearDynamic7 ==
  Wb : Inport
  Cr : Inport  Port=2
  motorT : Inport  Port=3
  ModelInit_RPM : Inport  Port=4
  PWM : Inport  Port=5
  Minimum Throttle Cutoff : simulink/Logic and Bit Operations/Compare To Constant  relop=>=  const=ModelParam_motorMinThr  OutDataTypeStr=uint8
  Motor_Dynamics : Subsystem  TreatAsAtomicUnit=on
  Motor_Dynamics_backup : StateSpace  Commented=on  A=-1/ModelParam_motorT  C=1/ModelParam_motorT  D=0  InitialCondition=ModelInit_RPM*ModelParam_motorT
  Product : Product
  Product1 : Product
  Signal_Saturation : Saturate  UpperLimit=0.95  LowerLimit=0
  Sum1 : Sum  Inputs=++|
  radW : Outport  VectorParamsAs1DForOutWhenUnconnected=off
  wires:
  PWM/1 -> Signal_Saturation/1
  Motor_Dynamics/1(motor_rate_act) -> radW/1
  Product/1 -> Motor_Dynamics/1(motor_rate_d)
  Signal_Saturation/1 -> Product1/2, Minimum Throttle Cutoff/1
  Product1/1 -> Sum1/2
  Sum1/1 -> Product/1
  Wb/1 -> Sum1/1
  Minimum Throttle Cutoff/1 -> Product/2
  Cr/1 -> Product1/1
  motorT/1 -> Motor_Dynamics/3(motorT)
  ModelInit_RPM/1 -> Motor_Dynamics/2(ModelInit_RPM)

== system Multicopter_vPC/Actuator Model: Motor_ESC/MotorNonlinearDynamic8 ==
  Wb : Inport
  Cr : Inport  Port=2
  motorT : Inport  Port=3
  ModelInit_RPM : Inport  Port=4
  PWM : Inport  Port=5
  Minimum Throttle Cutoff : simulink/Logic and Bit Operations/Compare To Constant  relop=>=  const=ModelParam_motorMinThr  OutDataTypeStr=uint8
  Motor_Dynamics : Subsystem  TreatAsAtomicUnit=on
  Motor_Dynamics_backup : StateSpace  Commented=on  A=-1/ModelParam_motorT  C=1/ModelParam_motorT  D=0  InitialCondition=ModelInit_RPM*ModelParam_motorT
  Product : Product
  Product1 : Product
  Signal_Saturation : Saturate  UpperLimit=0.95  LowerLimit=0
  Sum1 : Sum  Inputs=++|
  radW : Outport  VectorParamsAs1DForOutWhenUnconnected=off
  wires:
  ModelInit_RPM/1 -> Motor_Dynamics/2(ModelInit_RPM)
  motorT/1 -> Motor_Dynamics/3(motorT)
  Cr/1 -> Product1/1
  Minimum Throttle Cutoff/1 -> Product/2
  Wb/1 -> Sum1/1
  Sum1/1 -> Product/1
  Product1/1 -> Sum1/2
  Signal_Saturation/1 -> Minimum Throttle Cutoff/1, Product1/2
  Product/1 -> Motor_Dynamics/1(motor_rate_d)
  Motor_Dynamics/1(motor_rate_act) -> radW/1
  PWM/1 -> Signal_Saturation/1

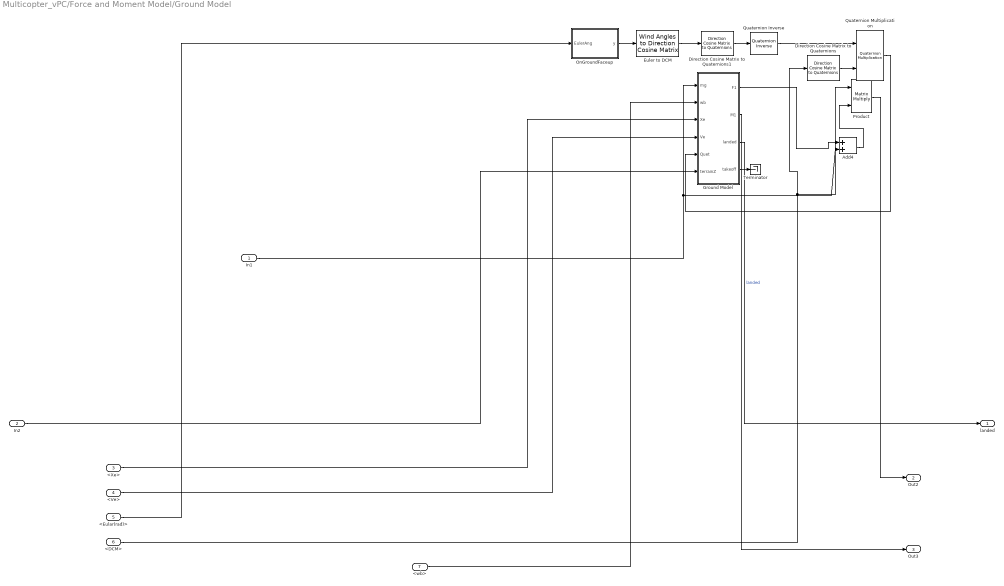
== system Multicopter_vPC/Force and Moment Model/Ground Model ==
  In1 : Inport
  In2 : Inport  Port=2
  <Xe> : Inport  Port=3
  <Ve> : Inport  Port=4
  <Eular(rad)> : Inport  Port=5
  <DCM> : Inport  Port=6
  <wb> : Inport  Port=7
  Add4 : Sum
  Direction Cosine Matrix to Quaternions : sharedtransform/Direction Cosine Matrix  to Quaternions  aMode=aMode  action=None  tolerance=eps(2)
      settings: SourceProductBaseCode=AE,PW,DR,MT,UV,VE
  Direction Cosine Matrix to Quaternions1 : sharedtransform/Direction Cosine Matrix  to Quaternions  aMode=aMode  action=None  tolerance=eps(2)
      settings: SourceProductBaseCode=AE,PW,DR,MT,UV,VE
  Euler to DCM : aerolibtransform2/Wind Angles to  Direction Cosine Matrix
      settings: SourceProductBaseCode=AE
  Ground Model : MATLAB Function  TreatAsAtomicUnit=on
  OnGroundFaceup : MATLAB Function  TreatAsAtomicUnit=on
  Product : Product  Multiplication=Matrix(*)
  Quaternion Inverse : aerolibutil/Quaternion Inverse
  Quaternion Multiplication : aerolibutil/Quaternion Multiplication
  Terminator : Terminator
  landed : Outport  VectorParamsAs1DForOutWhenUnconnected=off
  Out2 : Outport  Port=2  VectorParamsAs1DForOutWhenUnconnected=off
  Out3 : Outport  Port=3  VectorParamsAs1DForOutWhenUnconnected=off
  wires:
  <wb>/1 -> Ground Model/2(wb)
  OnGroundFaceup/1(y) -> Euler to DCM/1
  In2/1 -> Ground Model/6(terrainZ)
  Ground Model/3(landed) -> landed/1  "landed"
  Ground Model/1(F1) -> Add4/1
  Direction Cosine Matrix to Quaternions1/1 -> Quaternion Inverse/1
  Add4/1 -> Product/2
  Product/1 -> Out2/1
  Quaternion Multiplication/1 -> Ground Model/5(Quet)
  Euler to DCM/1 -> Direction Cosine Matrix to Quaternions1/1
  Ground Model/2(M1) -> Out3/1
  Quaternion Inverse/1 -> Quaternion Multiplication/1
  <DCM>/1 -> Product/1, Direction Cosine Matrix to Quaternions/1
  In1/1 -> Ground Model/1(mg), Add4/2
  Direction Cosine Matrix to Quaternions/1 -> Quaternion Multiplication/2
  Ground Model/4(takeoff) -> Terminator/1
  <Xe>/1 -> Ground Model/3(Xe)
  <Eular(rad)>/1 -> OnGroundFaceup/1(EulerAng)
  <Ve>/1 -> Ground Model/4(Ve)

== system Multicopter_vPC/Force and Moment Model/Propeller Model ==
  uavType : Inport
  MotorRads : Inport  Port=2
  uavR : Inport  Port=3
  uavDearo : Inport  Port=4
  Cm : Inport  Port=5
  Ct : Inport  Port=6
  Jm : Inport  Port=7
  wb : Inport  Port=8
  Vb : Inport  Port=9
  Cd : Inport  Port=10
  If : If  IfExpression=u1 >= 50
  Multicopter : Subsystem  TreatAsAtomicUnit=on
  Other Vehicle Types : Subsystem  TreatAsAtomicUnit=on
  Switch : Switch  Threshold=50
  Switch1 : Switch  Threshold=50
  Terminator : Terminator
  Terminator1 : Terminator
  Fb : Outport  VectorParamsAs1DForOutWhenUnconnected=off
  Mb : Outport  Port=2  VectorParamsAs1DForOutWhenUnconnected=off
  wires:
  Vb/1 -> Terminator/1
  Cd/1 -> Terminator1/1
  uavType/1 -> If/1, Switch/2, Switch1/2, Multicopter/1(uavType)
  Switch/1 -> Fb/1
  Switch1/1 -> Mb/1
  If/2 -> Multicopter/Action
  If/1 -> Other Vehicle Types/Action
  Other Vehicle Types/1(Fb) -> Switch/1
  Multicopter/1(Fb) -> Switch/3
  Other Vehicle Types/2(Mb) -> Switch1/1
  Multicopter/2(Mb) -> Switch1/3
  MotorRads/1 -> Other Vehicle Types/1(MotorRads), Multicopter/2(MotorRads)
  uavDearo/1 -> Multicopter/4(uavDearo)
  Cm/1 -> Multicopter/5(Cm)
  Ct/1 -> Multicopter/6(Ct)
  Jm/1 -> Multicopter/7(Jm)
  wb/1 -> Multicopter/8(wb)
  uavR/1 -> Multicopter/3(uavR)
